simulink model "dinamica_veiculo_ft"  (R2023a)
settings: Solver=VariableStepAuto  StartTime=0.0  StopTime=10.0  RelTol=1e-3
model workspace (MAT data in the model file):
  b = 50
  m = 1000
settings Model: Creator=Alexandre  LastModifiedBy=Alexandre

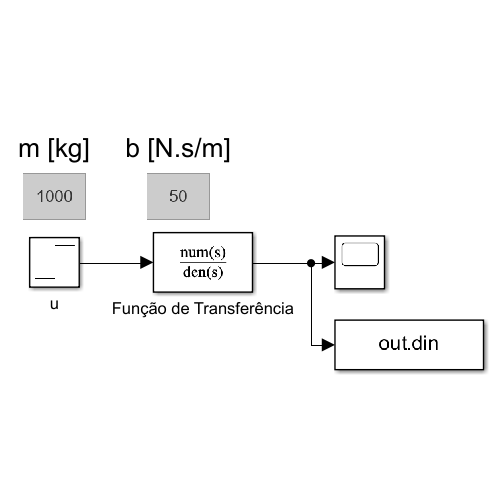
[thumbnail: Simulink's stored preview of the top-level diagram]
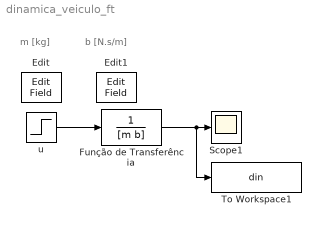
== system dinamica_veiculo_ft ==
  note: b [N.s/m]
  note: m [kg]
  Edit : EditField  LabelPosition=Hide  ShowInitialText=on  Alignment=Center
  Edit1 : EditField  LabelPosition=Hide  ShowInitialText=on  Alignment=Center
  Função de Transferência : TransferFcn  Denominator=[m b]
  Scope1 : Scope
  To Workspace1 : ToWorkspace  VariableName=din  SampleTime=-1
  u : Step  Time=0  After=500  SampleTime=0
  wires:
  u/1 -> Função de Transferência/1
  Função de Transferência/1 -> To Workspace1/1, Scope1/1
